simulink model "demo"  (R2021b)
settings: Solver=VariableStepAuto  StartTime=0.0  StopTime=10  RelTol=1e-3
undefined symbols (not defined in the file or in its folder): xc7vx485tffg1157
libraries: hdlBasic x1736, vmcUtilities x1
(part 7 of 7)

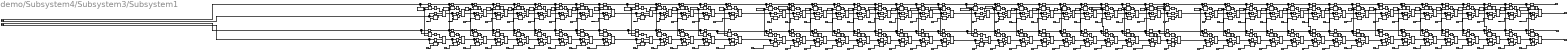
== system demo/Subsystem4/Subsystem3/Subsystem1 ==
  note: 50
  note: 80
  note: 70
  note: 60
  note: 40
  In1 : Inport
  In2 : Inport  Port=2
  In3 : Inport  Port=3
  In4 : Inport  Port=4
  In5 : Inport  Port=5
  In6 : Inport  Port=6
  In7 : Inport  Port=7
  In8 : Inport  Port=8
  In9 : Inport  Port=9
  In10 : Inport  Port=10
  In11 : Inport  Port=11
  In12 : Inport  Port=12
  In13 : Inport  Port=13
  In14 : Inport  Port=14
  In15 : Inport  Port=15
  In16 : Inport  Port=16
  In17 : Inport  Port=17
  In18 : Inport  Port=18
  In19 : Inport  Port=19
  In20 : Inport  Port=20
  In21 : Inport  Port=21
  In22 : Inport  Port=22
  In23 : Inport  Port=23
  In24 : Inport  Port=24
  In25 : Inport  Port=25
  In26 : Inport  Port=26
  In27 : Inport  Port=27
  In28 : Inport  Port=28
  In29 : Inport  Port=29
  In30 : Inport  Port=30
  In31 : Inport  Port=31
  In32 : Inport  Port=32
  In33 : Inport  Port=33
  In34 : Inport  Port=34
  In35 : Inport  Port=35
  In36 : Inport  Port=36
  In37 : Inport  Port=37
  In38 : Inport  Port=38
  In39 : Inport  Port=39
  In40 : Inport  Port=40
  In41 : Inport  Port=41
  In42 : Inport  Port=42
  In43 : Inport  Port=43
  In44 : Inport  Port=44
  In45 : Inport  Port=45
  In46 : Inport  Port=46
  In47 : Inport  Port=47
  In48 : Inport  Port=48
  In49 : Inport  Port=49
  In50 : Inport  Port=50
  In51 : Inport  Port=51
  In52 : Inport  Port=52
  In53 : Inport  Port=53
  In54 : Inport  Port=54
  In55 : Inport  Port=55
  In56 : Inport  Port=56
  In57 : Inport  Port=57
  In58 : Inport  Port=58
  In59 : Inport  Port=59
  In60 : Inport  Port=60
  In61 : Inport  Port=61
  In62 : Inport  Port=62
  In63 : Inport  Port=63
  In64 : Inport  Port=64
  In65 : Inport  Port=65
  In66 : Inport  Port=66
  In67 : Inport  Port=67
  In68 : Inport  Port=68
  In69 : Inport  Port=69
  In70 : Inport  Port=70
  In71 : Inport  Port=71
  In72 : Inport  Port=72
  In73 : Inport  Port=73
  In74 : Inport  Port=74
  In75 : Inport  Port=75
  In76 : Inport  Port=76
  In77 : Inport  Port=77
  In78 : Inport  Port=78
  In79 : Inport  Port=79
  In80 : Inport  Port=80
  In81 : Inport  Port=81
  In82 : Inport  Port=82
  In83 : Inport  Port=83
  In84 : Inport  Port=84
  In85 : Inport  Port=85
  In86 : Inport  Port=86
  In87 : Inport  Port=87
  In88 : Inport  Port=88
  In89 : Inport  Port=89
  In90 : Inport  Port=90
  In91 : Inport  Port=91
  In92 : Inport  Port=92
  In93 : Inport  Port=93
  In94 : Inport  Port=94
  In95 : Inport  Port=95
  In96 : Inport  Port=96
  In97 : Inport  Port=97
  In98 : Inport  Port=98
  In99 : Inport  Port=99
  In100 : Inport  Port=100
  In101 : Inport  Port=101
  In102 : Inport  Port=102
  AddSub{39..40,62..69,80..86,88..95,98..101,103,105..107,109,112,114..137,139,141..163,172..183,191,194,201} (98 alike) : hdlBasic/AddSub  mode=Addition  use_carryin=off  use_carryout=off  en=off  latency=1  precision=User Defined  arith_type="Signed  (2's comp)"  n_bits=32  bin_pt=0  quantization=Truncate  overflow=Wrap  use_behavioral_HDL=off  hw_selection=Fabric  pipelined=off  XmcBlockStatus=1  maskContainerNames=tabcontainer1  block_type=addsub  block_config=sysgen:Addsub_config
  Delay{110..113,177..180,182..184,186,191..192,195..196,199..200,202..204,207,209..214,217..218,220..221,224..226,229,235..236,239..240,242..243,245,247..248,251..255,293,295..296,298..299,302..303,305..306,308..309,311..313,315..316,318..319,323..324,326..327,329..330,332..333,335..338,340,342..343,345..347,350..351,353..354,357..358,360..362,364..365,367..369,371..373,375..376,379..380,383..384,386..387,389,402..404,409,413,419,429,433..434,437,446,448..449,451..453,455..456,458..459,461,463,465..466,468..469,472..474,476..477,479..480,482..485,487,506,517,519,531..532,534..535,538..539,541..542,544..545,548..550,553..554,556..558,560..561,563..564,566,568..569,571..572,574..575,578..580,582..583,585..586,588,590..591,593..594,596..597} (196 alike) : hdlBasic/Delay  rst=off  en=off  latency=1  reg_retiming=off  XmcBlockStatus=1  maskContainerNames=group1  block_type=delay  block_config=sysgen:Delay_config
  Delay{181,185,190,193,201,206,215,219,222..223,228,230,237,241,244,246,250,294,297,300..301,304,307,310,314,317,320,322,325,328,331,334,339,341,344,348..349,352,355..356,359,363,366,370,374,377..378,381..382,385,388,393,401,422,425,439,445,447,450,454,457,460,462,464,467,470..471,475,478,481,486,495,528,533,536..537,540,543,546..547,551..552,555,559,562,565,567,570,573,576..577,581,584,587,589,592,595,598} (98 alike) : hdlBasic/Delay  rst=off  en=off  latency=2  reg_retiming=off  XmcBlockStatus=1  maskContainerNames=group1  block_type=delay  block_config=sysgen:Delay_config
  Mux{38..39,58..67,78..85,87..92,95..96,98..105,110..117,119..136,139..158,161,170..180,183,190,194,198} (98 alike) : hdlBasic/Mux  inputs=2  en=off  latency=1  precision=Full  arith_type=Unsigned  n_bits=16  bin_pt=14  quantization=Truncate  overflow=Wrap  XmcBlockStatus=1  maskContainerNames=tabcontainer1  block_type=mux  block_config=sysgen:Mux_config
  Relational{37..38,60..69,79..85,87..92,95..96,98..100,102..106,111..118,120..122,124..137,140..163,174..183,185,192,196,201} (98 alike) : hdlBasic/Relational  mode=a>=b  op_type=Bool  en=off  latency=1  XmcBlockStatus=1  maskContainerNames=tabcontainer1  block_type=relational  block_config=sysgen:Relational_config
  logi_b36 : hdlBasic/Constant  const=-0.4193548387096773799598281584621872752904891967773437500  gui_display_data_type=Floating-point  arith_type=Floating-point  n_bits=8  bin_pt=8  preci_type=Double  exp_width=8  frac_width=24  explicit_period=on  period=1  XmcBlockStatus=1  maskContainerNames=tabcontainer1  block_type=constant  block_config=sysgen:Constant_config
  logi_b37 : hdlBasic/Constant  const=-0.4032258064516128781562542826577555388212203979492187500  gui_display_data_type=Floating-point  arith_type=Floating-point  n_bits=8  bin_pt=8  preci_type=Double  exp_width=8  frac_width=24  explicit_period=on  period=1  XmcBlockStatus=1  maskContainerNames=tabcontainer1  block_type=constant  block_config=sysgen:Constant_config
  logi_b38 : hdlBasic/Constant  const=-0.3870967741935483763526804068533238023519515991210937500  gui_display_data_type=Floating-point  arith_type=Floating-point  n_bits=8  bin_pt=8  preci_type=Double  exp_width=8  frac_width=24  explicit_period=on  period=1  XmcBlockStatus=1  maskContainerNames=tabcontainer1  block_type=constant  block_config=sysgen:Constant_config
  logi_b39 : hdlBasic/Constant  const=-0.3709677419354838745491065310488920658826828002929687500  gui_display_data_type=Floating-point  arith_type=Floating-point  n_bits=8  bin_pt=8  preci_type=Double  exp_width=8  frac_width=24  explicit_period=on  period=1  XmcBlockStatus=1  maskContainerNames=tabcontainer1  block_type=constant  block_config=sysgen:Constant_config
  logi_b40 : hdlBasic/Constant  const=-0.3548387096774193727455326552444603294134140014648437500  gui_display_data_type=Floating-point  arith_type=Floating-point  n_bits=8  bin_pt=8  preci_type=Double  exp_width=8  frac_width=24  explicit_period=on  period=1  XmcBlockStatus=1  maskContainerNames=tabcontainer1  block_type=constant  block_config=sysgen:Constant_config
  logi_b41 : hdlBasic/Constant  const=-0.3387096774193548154308075481822015717625617980957031250  gui_display_data_type=Floating-point  arith_type=Floating-point  n_bits=8  bin_pt=8  preci_type=Double  exp_width=8  frac_width=24  explicit_period=on  period=1  XmcBlockStatus=1  maskContainerNames=tabcontainer1  block_type=constant  block_config=sysgen:Constant_config
  logi_b42 : hdlBasic/Constant  const=-0.3225806451612903136272336723777698352932929992675781250  gui_display_data_type=Floating-point  arith_type=Floating-point  n_bits=8  bin_pt=8  preci_type=Double  exp_width=8  frac_width=24  explicit_period=on  period=1  XmcBlockStatus=1  maskContainerNames=tabcontainer1  block_type=constant  block_config=sysgen:Constant_config
  logi_b43 : hdlBasic/Constant  const=-0.3064516129032258118236597965733380988240242004394531250  gui_display_data_type=Floating-point  arith_type=Floating-point  n_bits=8  bin_pt=8  preci_type=Double  exp_width=8  frac_width=24  explicit_period=on  period=1  XmcBlockStatus=1  maskContainerNames=tabcontainer1  block_type=constant  block_config=sysgen:Constant_config
  logi_b44 : hdlBasic/Constant  const=-0.2903225806451612545089346895110793411731719970703125000  gui_display_data_type=Floating-point  arith_type=Floating-point  n_bits=8  bin_pt=8  preci_type=Double  exp_width=8  frac_width=24  explicit_period=on  period=1  XmcBlockStatus=1  maskContainerNames=tabcontainer1  block_type=constant  block_config=sysgen:Constant_config
  logi_b45 : hdlBasic/Constant  const=-0.2741935483870967527053608137066476047039031982421875000  gui_display_data_type=Floating-point  arith_type=Floating-point  n_bits=8  bin_pt=8  preci_type=Double  exp_width=8  frac_width=24  explicit_period=on  period=1  XmcBlockStatus=1  maskContainerNames=tabcontainer1  block_type=constant  block_config=sysgen:Constant_config
  logi_b46 : hdlBasic/Constant  const=-0.2580645161290322509017869379022158682346343994140625000  gui_display_data_type=Floating-point  arith_type=Floating-point  n_bits=8  bin_pt=8  preci_type=Double  exp_width=8  frac_width=24  explicit_period=on  period=1  XmcBlockStatus=1  maskContainerNames=tabcontainer1  block_type=constant  block_config=sysgen:Constant_config
  logi_b47 : hdlBasic/Constant  const=-0.2419354838709677490982130620977841317653656005859375000  gui_display_data_type=Floating-point  arith_type=Floating-point  n_bits=8  bin_pt=8  preci_type=Double  exp_width=8  frac_width=24  explicit_period=on  period=1  XmcBlockStatus=1  maskContainerNames=tabcontainer1  block_type=constant  block_config=sysgen:Constant_config
  logi_b48 : hdlBasic/Constant  const=-0.2258064516129032195390635706644388847053050994873046875  gui_display_data_type=Floating-point  arith_type=Floating-point  n_bits=8  bin_pt=8  preci_type=Double  exp_width=8  frac_width=24  explicit_period=on  period=1  XmcBlockStatus=1  maskContainerNames=tabcontainer1  block_type=constant  block_config=sysgen:Constant_config
  logi_b49 : hdlBasic/Constant  const=-0.2096774193548386899799140792310936376452445983886718750  gui_display_data_type=Floating-point  arith_type=Floating-point  n_bits=8  bin_pt=8  preci_type=Double  exp_width=8  frac_width=24  explicit_period=on  period=1  XmcBlockStatus=1  maskContainerNames=tabcontainer1  block_type=constant  block_config=sysgen:Constant_config
  logi_b50 : hdlBasic/Constant  const=-0.1935483870967741881763402034266619011759757995605468750  gui_display_data_type=Floating-point  arith_type=Floating-point  n_bits=8  bin_pt=8  preci_type=Double  exp_width=8  frac_width=24  explicit_period=on  period=1  XmcBlockStatus=1  maskContainerNames=tabcontainer1  block_type=constant  block_config=sysgen:Constant_config
  logi_b51 : hdlBasic/Constant  const=-0.1774193548387096863727663276222301647067070007324218750  gui_display_data_type=Floating-point  arith_type=Floating-point  n_bits=8  bin_pt=8  preci_type=Double  exp_width=8  frac_width=24  explicit_period=on  period=1  XmcBlockStatus=1  maskContainerNames=tabcontainer1  block_type=constant  block_config=sysgen:Constant_config
  logi_b52 : hdlBasic/Constant  const=-0.1612903225806451568136168361888849176466464996337890625  gui_display_data_type=Floating-point  arith_type=Floating-point  n_bits=8  bin_pt=8  preci_type=Double  exp_width=8  frac_width=24  explicit_period=on  period=1  XmcBlockStatus=1  maskContainerNames=tabcontainer1  block_type=constant  block_config=sysgen:Constant_config
  logi_b53 : hdlBasic/Constant  const=-0.1451612903225806272544673447555396705865859985351562500  gui_display_data_type=Floating-point  arith_type=Floating-point  n_bits=8  bin_pt=8  preci_type=Double  exp_width=8  frac_width=24  explicit_period=on  period=1  XmcBlockStatus=1  maskContainerNames=tabcontainer1  block_type=constant  block_config=sysgen:Constant_config
  logi_b54 : hdlBasic/Constant  const=-0.1290322580645161254508934689511079341173171997070312500  gui_display_data_type=Floating-point  arith_type=Floating-point  n_bits=8  bin_pt=8  preci_type=Double  exp_width=8  frac_width=24  explicit_period=on  period=1  XmcBlockStatus=1  maskContainerNames=tabcontainer1  block_type=constant  block_config=sysgen:Constant_config
  logi_b55 : hdlBasic/Constant  const=-0.1129032258064516097695317853322194423526525497436523438  gui_display_data_type=Floating-point  arith_type=Floating-point  n_bits=8  bin_pt=8  preci_type=Double  exp_width=8  frac_width=24  explicit_period=on  period=1  XmcBlockStatus=1  maskContainerNames=tabcontainer1  block_type=constant  block_config=sysgen:Constant_config
  logi_b56 : hdlBasic/Constant  const=-0.0967741935483870940881701017133309505879878997802734375  gui_display_data_type=Floating-point  arith_type=Floating-point  n_bits=8  bin_pt=8  preci_type=Double  exp_width=8  frac_width=24  explicit_period=on  period=1  XmcBlockStatus=1  maskContainerNames=tabcontainer1  block_type=constant  block_config=sysgen:Constant_config
  logi_b57 : hdlBasic/Constant  const=-0.0806451612903225784068084180944424588233232498168945312  gui_display_data_type=Floating-point  arith_type=Floating-point  n_bits=8  bin_pt=8  preci_type=Double  exp_width=8  frac_width=24  explicit_period=on  period=1  XmcBlockStatus=1  maskContainerNames=tabcontainer1  block_type=constant  block_config=sysgen:Constant_config
  logi_b58 : hdlBasic/Constant  const=-0.0645161290322580627254467344755539670586585998535156250  gui_display_data_type=Floating-point  arith_type=Floating-point  n_bits=8  bin_pt=8  preci_type=Double  exp_width=8  frac_width=24  explicit_period=on  period=1  XmcBlockStatus=1  maskContainerNames=tabcontainer1  block_type=constant  block_config=sysgen:Constant_config
  logi_b59 : hdlBasic/Constant  const=-0.0483870967741935470440850508566654752939939498901367188  gui_display_data_type=Floating-point  arith_type=Floating-point  n_bits=8  bin_pt=8  preci_type=Double  exp_width=8  frac_width=24  explicit_period=on  period=1  XmcBlockStatus=1  maskContainerNames=tabcontainer1  block_type=constant  block_config=sysgen:Constant_config
  logi_b60 : hdlBasic/Constant  const=-0.0322580645161290313627233672377769835293292999267578125  gui_display_data_type=Floating-point  arith_type=Floating-point  n_bits=8  bin_pt=8  preci_type=Double  exp_width=8  frac_width=24  explicit_period=on  period=1  XmcBlockStatus=1  maskContainerNames=tabcontainer1  block_type=constant  block_config=sysgen:Constant_config
  logi_b61 : hdlBasic/Constant  const=-0.0161290322580645156813616836188884917646646499633789062  gui_display_data_type=Floating-point  arith_type=Floating-point  n_bits=8  bin_pt=8  preci_type=Double  exp_width=8  frac_width=24  explicit_period=on  period=1  XmcBlockStatus=1  maskContainerNames=tabcontainer1  block_type=constant  block_config=sysgen:Constant_config
  logi_b62 : hdlBasic/Constant  const=0.0000000000000000000000000000000000000000000000000000000  gui_display_data_type=Floating-point  arith_type=Floating-point  n_bits=8  bin_pt=8  preci_type=Double  exp_width=8  frac_width=24  explicit_period=on  period=1  XmcBlockStatus=1  maskContainerNames=tabcontainer1  block_type=constant  block_config=sysgen:Constant_config
  logi_b63 : hdlBasic/Constant  const=0.0161290322580645156813616836188884917646646499633789062  gui_display_data_type=Floating-point  arith_type=Floating-point  n_bits=8  bin_pt=8  preci_type=Double  exp_width=8  frac_width=24  explicit_period=on  period=1  XmcBlockStatus=1  maskContainerNames=tabcontainer1  block_type=constant  block_config=sysgen:Constant_config
  logi_b64 : hdlBasic/Constant  const=0.0322580645161290313627233672377769835293292999267578125  gui_display_data_type=Floating-point  arith_type=Floating-point  n_bits=8  bin_pt=8  preci_type=Double  exp_width=8  frac_width=24  explicit_period=on  period=1  XmcBlockStatus=1  maskContainerNames=tabcontainer1  block_type=constant  block_config=sysgen:Constant_config
  logi_b65 : hdlBasic/Constant  const=0.0483870967741935470440850508566654752939939498901367188  gui_display_data_type=Floating-point  arith_type=Floating-point  n_bits=8  bin_pt=8  preci_type=Double  exp_width=8  frac_width=24  explicit_period=on  period=1  XmcBlockStatus=1  maskContainerNames=tabcontainer1  block_type=constant  block_config=sysgen:Constant_config
  logi_b66 : hdlBasic/Constant  const=0.0645161290322580627254467344755539670586585998535156250  gui_display_data_type=Floating-point  arith_type=Floating-point  n_bits=8  bin_pt=8  preci_type=Double  exp_width=8  frac_width=24  explicit_period=on  period=1  XmcBlockStatus=1  maskContainerNames=tabcontainer1  block_type=constant  block_config=sysgen:Constant_config
  logi_b67 : hdlBasic/Constant  const=0.0806451612903225784068084180944424588233232498168945312  gui_display_data_type=Floating-point  arith_type=Floating-point  n_bits=8  bin_pt=8  preci_type=Double  exp_width=8  frac_width=24  explicit_period=on  period=1  XmcBlockStatus=1  maskContainerNames=tabcontainer1  block_type=constant  block_config=sysgen:Constant_config
  logi_b68 : hdlBasic/Constant  const=0.0967741935483870940881701017133309505879878997802734375  gui_display_data_type=Floating-point  arith_type=Floating-point  n_bits=8  bin_pt=8  preci_type=Double  exp_width=8  frac_width=24  explicit_period=on  period=1  XmcBlockStatus=1  maskContainerNames=tabcontainer1  block_type=constant  block_config=sysgen:Constant_config
  logi_b69 : hdlBasic/Constant  const=0.1129032258064516097695317853322194423526525497436523438  gui_display_data_type=Floating-point  arith_type=Floating-point  n_bits=8  bin_pt=8  preci_type=Double  exp_width=8  frac_width=24  explicit_period=on  period=1  XmcBlockStatus=1  maskContainerNames=tabcontainer1  block_type=constant  block_config=sysgen:Constant_config
  logi_b70 : hdlBasic/Constant  const=0.1290322580645161254508934689511079341173171997070312500  gui_display_data_type=Floating-point  arith_type=Floating-point  n_bits=8  bin_pt=8  preci_type=Double  exp_width=8  frac_width=24  explicit_period=on  period=1  XmcBlockStatus=1  maskContainerNames=tabcontainer1  block_type=constant  block_config=sysgen:Constant_config
  logi_b71 : hdlBasic/Constant  const=0.1451612903225806272544673447555396705865859985351562500  gui_display_data_type=Floating-point  arith_type=Floating-point  n_bits=8  bin_pt=8  preci_type=Double  exp_width=8  frac_width=24  explicit_period=on  period=1  XmcBlockStatus=1  maskContainerNames=tabcontainer1  block_type=constant  block_config=sysgen:Constant_config
  logi_b72 : hdlBasic/Constant  const=0.1612903225806451568136168361888849176466464996337890625  gui_display_data_type=Floating-point  arith_type=Floating-point  n_bits=8  bin_pt=8  preci_type=Double  exp_width=8  frac_width=24  explicit_period=on  period=1  XmcBlockStatus=1  maskContainerNames=tabcontainer1  block_type=constant  block_config=sysgen:Constant_config
  logi_b73 : hdlBasic/Constant  const=0.1774193548387096863727663276222301647067070007324218750  gui_display_data_type=Floating-point  arith_type=Floating-point  n_bits=8  bin_pt=8  preci_type=Double  exp_width=8  frac_width=24  explicit_period=on  period=1  XmcBlockStatus=1  maskContainerNames=tabcontainer1  block_type=constant  block_config=sysgen:Constant_config
  logi_b74 : hdlBasic/Constant  const=0.1935483870967741881763402034266619011759757995605468750  gui_display_data_type=Floating-point  arith_type=Floating-point  n_bits=8  bin_pt=8  preci_type=Double  exp_width=8  frac_width=24  explicit_period=on  period=1  XmcBlockStatus=1  maskContainerNames=tabcontainer1  block_type=constant  block_config=sysgen:Constant_config
  logi_b75 : hdlBasic/Constant  const=0.2096774193548386899799140792310936376452445983886718750  gui_display_data_type=Floating-point  arith_type=Floating-point  n_bits=8  bin_pt=8  preci_type=Double  exp_width=8  frac_width=24  explicit_period=on  period=1  XmcBlockStatus=1  maskContainerNames=tabcontainer1  block_type=constant  block_config=sysgen:Constant_config
  logi_b76 : hdlBasic/Constant  const=0.2258064516129032195390635706644388847053050994873046875  gui_display_data_type=Floating-point  arith_type=Floating-point  n_bits=8  bin_pt=8  preci_type=Double  exp_width=8  frac_width=24  explicit_period=on  period=1  XmcBlockStatus=1  maskContainerNames=tabcontainer1  block_type=constant  block_config=sysgen:Constant_config
  logi_b77 : hdlBasic/Constant  const=0.2419354838709677490982130620977841317653656005859375000  gui_display_data_type=Floating-point  arith_type=Floating-point  n_bits=8  bin_pt=8  preci_type=Double  exp_width=8  frac_width=24  explicit_period=on  period=1  XmcBlockStatus=1  maskContainerNames=tabcontainer1  block_type=constant  block_config=sysgen:Constant_config
  logi_b78 : hdlBasic/Constant  const=0.2580645161290322509017869379022158682346343994140625000  gui_display_data_type=Floating-point  arith_type=Floating-point  n_bits=8  bin_pt=8  preci_type=Double  exp_width=8  frac_width=24  explicit_period=on  period=1  XmcBlockStatus=1  maskContainerNames=tabcontainer1  block_type=constant  block_config=sysgen:Constant_config
  logi_b79 : hdlBasic/Constant  const=0.2741935483870967527053608137066476047039031982421875000  gui_display_data_type=Floating-point  arith_type=Floating-point  n_bits=8  bin_pt=8  preci_type=Double  exp_width=8  frac_width=24  explicit_period=on  period=1  XmcBlockStatus=1  maskContainerNames=tabcontainer1  block_type=constant  block_config=sysgen:Constant_config
  logi_b80 : hdlBasic/Constant  const=0.2903225806451612545089346895110793411731719970703125000  gui_display_data_type=Floating-point  arith_type=Floating-point  n_bits=8  bin_pt=8  preci_type=Double  exp_width=8  frac_width=24  explicit_period=on  period=1  XmcBlockStatus=1  maskContainerNames=tabcontainer1  block_type=constant  block_config=sysgen:Constant_config
  logi_b81 : hdlBasic/Constant  const=0.3064516129032258118236597965733380988240242004394531250  gui_display_data_type=Floating-point  arith_type=Floating-point  n_bits=8  bin_pt=8  preci_type=Double  exp_width=8  frac_width=24  explicit_period=on  period=1  XmcBlockStatus=1  maskContainerNames=tabcontainer1  block_type=constant  block_config=sysgen:Constant_config
  logi_b82 : hdlBasic/Constant  const=0.3225806451612903136272336723777698352932929992675781250  gui_display_data_type=Floating-point  arith_type=Floating-point  n_bits=8  bin_pt=8  preci_type=Double  exp_width=8  frac_width=24  explicit_period=on  period=1  XmcBlockStatus=1  maskContainerNames=tabcontainer1  block_type=constant  block_config=sysgen:Constant_config
  logi_b83 : hdlBasic/Constant  const=0.3387096774193548154308075481822015717625617980957031250  gui_display_data_type=Floating-point  arith_type=Floating-point  n_bits=8  bin_pt=8  preci_type=Double  exp_width=8  frac_width=24  explicit_period=on  period=1  XmcBlockStatus=1  maskContainerNames=tabcontainer1  block_type=constant  block_config=sysgen:Constant_config
  logi_b84 : hdlBasic/Constant  const=0.3548387096774193727455326552444603294134140014648437500  gui_display_data_type=Floating-point  arith_type=Floating-point  n_bits=8  bin_pt=8  preci_type=Double  exp_width=8  frac_width=24  explicit_period=on  period=1  XmcBlockStatus=1  maskContainerNames=tabcontainer1  block_type=constant  block_config=sysgen:Constant_config
  Out1 : Outport
  Out2 : Outport  Port=2
  Out3 : Outport  Port=3
  Out4 : Outport  Port=4
  wires:
  In12/1 -> AddSub86/2
  Delay361/1 -> Mux154/1
  Delay112/1 -> Mux38/1
  Delay590/1 -> Mux115/1
  Delay384/1 -> Mux147/2
  Delay213/1 -> Mux111/2
  AddSub67/1 -> Mux65/3
  Delay329/1 -> Mux78/1
  Relational135/1 -> Delay571/1
  Relational113/1 -> Delay582/1
  AddSub131/1 -> Mux129/3
  Delay245/1 -> Mux194/2
  Delay313/1 -> Mux63/2
  Relational117/1 -> Delay596/1
  AddSub112/1 -> Mux59/3
  Delay326/1 -> Mux67/1
  In71/1 -> AddSub95/2
  Relational102/1 -> Delay448/1
  Delay368/1 -> Mux156/2
  Delay531/1 -> Mux121/1
  Relational79/1 -> Delay295/1
  Relational196/1 -> Delay473/1
  Relational112/1 -> Delay224/1
  Mux131/1 -> AddSub132/1, Delay564/1
  Mux116/1 -> AddSub131/1, Delay597/1
  Delay382/1 -> Delay393/1, Relational163/1
  Relational131/1 -> Delay548/1
  logi_b66/1 -> Relational120/2, Relational137/2
  Mux61/1 -> AddSub91/1, Delay218/1
  Mux140/1 -> Delay333/1, AddSub145/1
  Delay336/1 -> Mux96/1
  Delay462/1 -> Relational122/1, Delay495/1
  Mux65/1 -> AddSub68/1, Delay324/1
  logi_b37/1 -> Relational62/2, Relational68/2
  Delay306/1 -> Mux83/2
  logi_b72/1 -> Relational148/2, Relational156/2
  logi_b83/1 -> Relational183/2, Relational106/2
  Relational201/1 -> Delay433/1
  In49/1 -> AddSub132/2
  Delay593/1 -> Mux116/1
  In2/1 -> Delay184/1, AddSub112/1
  Delay349/1 -> Relational152/1, Delay382/1
  Delay542/1 -> Mux124/2
  AddSub151/1 -> Mux147/3
  Relational158/1 -> Delay364/1
  Delay569/1 -> Mux133/2
  logi_b58/1 -> Relational98/2, Relational122/2
  Delay315/1 -> Mux64/1
  Delay479/1 -> Mux177/1
  Delay482/1 -> Mux178/1
  Mux141/1 -> Delay337/1, AddSub162/1
  In8/1 -> AddSub109/2
  In20/1 -> AddSub100/2
  AddSub162/1 -> Mux96/3
  logi_b40/1 -> Relational65/2, Relational81/2
  AddSub114/1 -> Mux111/3
  Delay301/1 -> Delay304/1, Relational82/1
  logi_b45/1 -> Relational89/2, Relational88/2
  Delay583/1 -> Mux113/2
  Delay214/1 -> Mux61/2
  AddSub105/1 -> Mux131/3
  In30/1 -> AddSub101/2
  Delay447/1 -> Delay450/1, Relational103/1
  Mux62/1 -> AddSub65/1, Delay313/1
  AddSub128/1 -> Mux139/3
  Relational82/1 -> Delay305/1
  In22/1 -> AddSub172/2
  Mux80/1 -> AddSub81/1, Delay299/1
  Delay439/1 -> Relational196/1, Delay462/1
  Mux98/1 -> AddSub100/1, Delay221/1
  logi_b43/1 -> Relational69/2, Relational84/2
  Delay222/1 -> Delay547/1, Relational37/1
  AddSub159/1 -> Mux157/3
  Delay203/1 -> Mux58/1
  Delay592/1 -> Delay595/1, Relational117/1
  Delay314/1 -> Relational63/1, Delay317/1
  Delay481/1 -> Relational162/1, Delay486/1
  Delay464/1 -> Relational177/1, Delay467/1
  AddSub129/1 -> Mux126/3
  Delay218/1 -> Mux98/2
  Mux88/1 -> Delay204/1, AddSub109/1
  Relational181/1 -> Delay479/1
  Relational160/1 -> Delay345/1
  Delay344/1 -> Delay464/1, Relational176/1
  Mux66/1 -> AddSub69/1, Delay327/1
  Delay594/1 -> Mux116/2
  Relational149/1 -> Delay383/1
  Relational114/1 -> Delay585/1
  AddSub121/1 -> Mux119/3
  Relational174/1 -> Delay429/1
  AddSub173/1 -> Mux180/3
  Delay551/1 -> Relational111/1, Delay223/1
  Delay571/1 -> Mux134/1
  logi_b39/1 -> Relational64/2, Relational80/2
  Delay300/1 -> Delay301/1, Relational81/1
  Delay486/1 -> Out3/1
  Mux125/1 -> AddSub129/1, Delay549/1
  Delay413/1 -> Mux150/2
  Relational140/1 -> Delay252/1
  AddSub134/1 -> Mux133/3
  Mux110/1 -> AddSub144/1, Delay351/1
  Delay239/1 -> Mux91/1
  Mux177/1 -> AddSub181/1, Delay483/1
  Delay403/1 -> Mux103/2
  Delay589/1 -> Delay592/1, Relational116/1
  logi_b50/1 -> Relational121/2, Relational95/2
  Relational133/1 -> Delay563/1
  Delay595/1 -> Relational120/1, Delay598/1
  Relational62/1 -> Delay182/1
  In34/1 -> AddSub161/2
  In72/1 -> AddSub39/2
  Delay235/1 -> Mux194/1
  Mux123/1 -> AddSub126/1, Delay542/1
  logi_b84/1 -> Relational162/2, Relational175/2
  In57/1 -> AddSub88/2
  Relational68/1 -> Delay186/1
  Mux179/1 -> Out2/1
  Mux87/1 -> Delay200/1, AddSub92/1
  AddSub100/1 -> Mux99/3
  AddSub109/1 -> Mux58/3
  AddSub117/1 -> Mux114/3
  Relational103/1 -> Delay452/1
  Mux58/1 -> AddSub90/1, Delay214/1
  Relational122/1 -> Delay506/1
  AddSub65/1 -> Mux63/3
  Delay355/1 -> Delay356/1, Relational156/1
  In21/1 -> AddSub40/2
  Relational92/1 -> Delay242/1
  AddSub181/1 -> Mux178/3
  Delay251/1 -> Mux128/1
  AddSub126/1 -> Mux124/3
  Delay365/1 -> Mux155/2
  AddSub148/1 -> Mux145/3
  Delay337/1 -> Mux96/2
  Delay434/1 -> Mux161/2
  Delay113/1 -> Mux38/2
  Delay199/1 -> Mux89/1
  Delay409/1 -> Mux180/1
  Delay597/1 -> Mux129/2
  Relational80/1 -> Delay298/1
  logi_b77/1 -> Relational176/2, Relational182/2
  AddSub176/1 -> Mux174/3
  Delay200/1 -> Mux89/2
  Delay110/1 -> Mux39/1
  Delay574/1 -> Mux135/1
  AddSub98/1 -> Mux95/3
  logi_b74/1 -> Relational150/2, Relational158/2
  logi_b44/1 -> Relational85/2, Relational87/2
  AddSub172/1 -> Mux183/3
  In98/1 -> AddSub117/2
  AddSub135/1 -> Mux134/3
  Delay206/1 -> Delay215/1, Relational96/1
  In90/1 -> AddSub118/2
  AddSub141/1 -> Mux140/3
  Delay554/1 -> Mux119/2
  Relational180/1 -> Delay476/1
  Delay372/1 -> Mux144/1
  Mux114/1 -> AddSub118/1, Delay591/1
  Delay331/1 -> Relational85/1, Delay193/1
  Delay202/1 -> Mux90/1
  Delay250/1 -> Relational144/1, Delay334/1
  Mux143/1 -> AddSub147/1, Delay373/1
  Delay577/1 -> Relational130/1, Delay230/1
  In46/1 -> AddSub120/2
  AddSub174/1 -> Mux171/3
  Delay332/1 -> Mux142/1
  Mux95/1 -> AddSub99/1, Delay209/1
  Delay584/1 -> Relational114/1, Delay587/1
  Delay586/1 -> Mux114/2
  In80/1 -> AddSub129/2
  Mux153/1 -> AddSub156/1, Delay362/1
  In38/1 -> AddSub156/2
  AddSub132/1 -> Mux132/3
  Mux161/1 -> AddSub161/1, Delay451/1
  AddSub139/1 -> Mux150/3
  Delay453/1 -> Mux100/2
  Mux124/1 -> AddSub127/1, Delay545/1
  Delay244/1 -> Relational38/1, Delay552/1
  In62/1 -> AddSub68/2
  Delay246/1 -> Relational143/1, Delay339/1
  AddSub158/1 -> Mux156/3
  logi_b82/1 -> Relational181/2, Relational104/2
  logi_b69/1 -> Relational145/2, Relational151/2
  Mux135/1 -> AddSub137/1, Delay579/1
  Delay560/1 -> Mux131/1
  Delay575/1 -> Mux135/2
  Mux83/1 -> AddSub85/1, Delay309/1
  Relational146/1 -> Delay372/1
  Mux112/1 -> AddSub116/1, Delay583/1
  Mux127/1 -> Delay226/1, AddSub194/1
  Delay598/1 -> Relational140/1, Delay250/1
  Mux81/1 -> AddSub83/1, Delay303/1
  Delay325/1 -> Delay328/1, Relational67/1
  Relational106/1 -> Delay458/1
  logi_b80/1 -> Relational179/2, Relational102/2
  Delay506/1 -> Mux127/1
  AddSub149/1 -> Mux146/3
  Delay327/1 -> Mux67/2
  Delay219/1 -> Relational100/1, Delay222/1
  Delay385/1 -> Relational153/1, Delay388/1
  In43/1 -> AddSub155/2
  In7/1 -> AddSub62/2
  Delay353/1 -> Mux152/1
  Delay587/1 -> Delay589/1, Relational115/1
  Delay561/1 -> Mux131/2
  In11/1 -> AddSub85/2
  Relational185/1 -> Delay446/1
  Delay322/1 -> Delay325/1, Relational66/1
  Delay581/1 -> Relational113/1, Delay584/1
  In51/1 -> AddSub153/2
  Mux174/1 -> AddSub177/1, Delay474/1
  Mux113/1 -> AddSub117/1, Delay586/1
  Delay335/1 -> Mux143/1
  In56/1 -> AddSub82/2
  logi_b68/1 -> Relational144/2, Relational143/2
  Delay483/1 -> Mux178/2
  In9/1 -> AddSub90/2
  AddSub90/1 -> Mux61/3
  Delay573/1 -> Relational137/1, Delay576/1
  In14/1 -> AddSub103/2
  Mux64/1 -> AddSub67/1, Delay319/1
  In73/1 -> AddSub121/2
  logi_b46/1 -> Relational90/2, Relational96/2
  Relational61/1 -> Delay179/1
  In41/1 -> AddSub139/2
  logi_b62/1 -> Relational114/2, Relational133/2
  Delay422/1 -> Delay439/1, Relational185/1
  Delay341/1 -> Delay401/1, Relational182/1
  Delay539/1 -> Mux123/2
  Relational143/1 -> Delay336/1
  Delay317/1 -> Relational64/1, Delay320/1
  Delay333/1 -> Mux142/2
  AddSub88/1 -> Mux87/3
  logi_b48/1 -> Relational92/2, Relational100/2
  Delay375/1 -> Mux145/1
  Relational84/1 -> Delay311/1
  Relational38/1 -> Delay112/1
  In42/1 -> AddSub134/2
  In39/1 -> AddSub157/2
  In102/1 -> AddSub148/2
  logi_b56/1 -> Relational129/2, Relational185/2
  AddSub183/1 -> Mux194/3
  logi_b54/1 -> Relational127/2, Relational163/2
  In6/1 -> AddSub112/2
  In58/1 -> AddSub178/2
  Relational152/1 -> Delay360/1
  AddSub68/1 -> Mux66/3
  Delay351/1 -> Mux151/2
  Relational85/1 -> Delay195/1
  AddSub150/1 -> Mux161/3
  Mux39/1 -> Delay566/1, AddSub98/1
  In60/1 -> AddSub181/2
  In77/1 -> AddSub176/2
  Delay465/1 -> Mux173/1
  In96/1 -> AddSub115/2
  Mux152/1 -> AddSub155/1, Delay358/1
  Delay111/1 -> Mux39/2
  In25/1 -> AddSub160/2
  Mux170/1 -> AddSub173/1, Delay419/1
  Delay459/1 -> Mux102/2
  In84/1 -> AddSub133/2
  Delay550/1 -> Mux127/2
  Mux151/1 -> AddSub153/1, Delay354/1
  Delay297/1 -> Relational80/1, Delay300/1
  Delay253/1 -> Mux140/2
  Delay389/1 -> Mux170/2
  Delay495/1 -> Relational105/1, Delay228/1
  Delay377/1 -> Delay378/1, Relational148/1
  Delay298/1 -> Mux81/1
  Delay556/1 -> Mux120/1
  In35/1 -> AddSub135/2
  AddSub137/1 -> Mux136/3
  Mux149/1 -> AddSub159/1, Delay346/1
  Delay477/1 -> Mux176/2
  Relational163/1 -> Delay404/1
  Relational148/1 -> Delay379/1
  Mux92/1 -> AddSub39/1, Delay113/1
  In89/1 -> AddSub125/2
  Delay220/1 -> Mux99/1
  Relational63/1 -> Delay315/1
  AddSub178/1 -> Mux176/3
  AddSub136/1 -> Mux135/3
  In44/1 -> AddSub98/2
  Relational64/1 -> Delay318/1
  Delay180/1 -> Mux62/2
  In92/1 -> AddSub122/2
  Relational95/1 -> Delay557/1
  Relational156/1 -> Delay357/1
  In13/1 -> AddSub201/2
  Delay472/1 -> Mux175/1
  Delay196/1 -> Mux87/2
  Mux172/1 -> AddSub172/1, Delay484/1
  Relational151/1 -> Delay340/1
  Delay461/1 -> Mux179/1
  Mux60/1 -> AddSub63/1, Delay296/1
  Relational66/1 -> Delay326/1
  Mux122/1 -> AddSub125/1, Delay539/1
  Delay532/1 -> Mux121/2
  logi_b59/1 -> Relational111/2, Relational105/2
  In5/1 -> AddSub182/2
  Delay404/1 -> Mux150/1
  Delay252/1 -> Mux140/1
  In74/1 -> AddSub159/2
  AddSub82/1 -> Mux79/3
  AddSub94/1 -> Mux91/3
  Delay469/1 -> Mux174/2
  In32/1 -> AddSub143/2
  In78/1 -> AddSub126/2
  AddSub142/1 -> Mux141/3
  Delay562/1 -> Relational133/1, Delay565/1
  Delay241/1 -> Relational92/1, Delay244/1
  In65/1 -> AddSub65/2
  Delay295/1 -> Mux80/1
  logi_b73/1 -> Relational149/2, Relational157/2
  AddSub155/1 -> Mux153/3
  In53/1 -> Delay180/1, AddSub64/1
  AddSub106/1 -> Mux102/3
  Relational127/1 -> Delay538/1
  Mux82/1 -> AddSub84/1, Delay306/1
  Delay540/1 -> Delay543/1, Relational129/1
  logi_b71/1 -> Relational147/2, Relational155/2
  Relational183/1 -> Delay482/1
  logi_b67/1 -> Relational140/2, Relational142/2
  AddSub133/1 -> Mux130/3
  AddSub115/1 -> Mux112/3
  Delay537/1 -> Delay540/1, Relational128/1
  AddSub39/1 -> Mux38/3
  In24/1 -> AddSub142/2
  Delay191/1 -> Mux88/1
  In94/1 -> AddSub124/2
  Delay572/1 -> Mux134/2
  Relational125/1 -> Delay531/1
  In100/1 -> AddSub146/2
  Mux96/1 -> AddSub143/1, Delay347/1
  Delay401/1 -> Relational192/1, Delay425/1
  Mux119/1 -> AddSub122/1, Delay517/1
  Mux130/1 -> AddSub141/1, Delay253/1
  In37/1 -> AddSub137/2
  Mux146/1 -> AddSub151/1, Delay384/1
  Delay545/1 -> Mux125/2
  In1/1 -> Relational60/1, Delay185/1
  Mux190/1 -> AddSub191/1, Delay449/1
  In69/1 -> AddSub93/2
  Delay480/1 -> Mux177/2
  Delay433/1 -> Mux190/1
  Delay237/1 -> Relational91/1, Delay241/1
  In79/1 -> AddSub127/2
  Delay179/1 -> Mux62/1
  Delay183/1 -> Mux59/1
  Delay299/1 -> Mux81/2
  logi_b57/1 -> Relational131/2, Relational196/2
  In15/1 -> AddSub83/2
  Delay582/1 -> Mux113/1
  Delay363/1 -> Relational159/1, Delay366/1
  Delay294/1 -> Relational79/1, Delay297/1
  In91/1 -> AddSub149/2
  Relational111/1 -> Delay212/1
  Delay538/1 -> Mux123/1
  Mux180/1 -> AddSub180/1, Delay437/1
  Relational162/1 -> Delay402/1
  In40/1 -> AddSub158/2
  Delay445/1 -> Delay447/1, Relational102/1
  AddSub152/1 -> Mux148/3
  logi_b63/1 -> Relational115/2, Relational134/2
  AddSub123/1 -> Mux121/3
  Delay476/1 -> Mux176/1
  Delay217/1 -> Mux98/1
  Mux111/1 -> AddSub115/1, Delay580/1
  Mux176/1 -> AddSub179/1, Delay480/1
  Mux67/1 -> AddSub80/1, Delay330/1
  Relational128/1 -> Delay541/1
  Mux103/1 -> Out4/1
  In26/1 -> AddSub163/2
  Relational100/1 -> Delay220/1
  Relational81/1 -> Delay302/1
  Relational182/1 -> Delay519/1
  Delay186/1 -> Mux60/1
  Delay552/1 -> Delay555/1, Relational121/1
  Delay470/1 -> Delay471/1, Relational179/1
  Delay185/1 -> Delay294/1, Relational68/1
  Mux144/1 -> AddSub148/1, Delay376/1
  In76/1 -> AddSub175/2
  Relational60/1 -> Delay183/1
  Delay467/1 -> Relational178/1, Delay470/1
  In68/1 -> AddSub92/2
  Relational175/1 -> Delay461/1
  Delay579/1 -> Mux136/2
  logi_b60/1 -> Relational112/2, Relational118/2
  Delay449/1 -> Mux198/2
  Delay318/1 -> Mux65/1
  Delay568/1 -> Mux133/1
  Delay388/1 -> Relational160/1, Delay344/1
  Relational118/1 -> Delay229/1
  In95/1 -> AddSub114/2
  AddSub119/1 -> Mux116/3
  AddSub201/1 -> Mux100/3
  logi_b55/1 -> Relational128/2, Relational174/2
  Mux100/1 -> AddSub103/1, Delay456/1
  Relational132/1 -> Delay560/1
  Mux120/1 -> AddSub123/1, Delay532/1
  logi_b52/1 -> Relational125/2, Relational141/2
  Relational37/1 -> Delay110/1
  AddSub177/1 -> Mux175/3
  Mux139/1 -> AddSub139/1, Delay413/1
  AddSub99/1 -> Mux117/3
  In63/1 -> AddSub177/2
  Delay309/1 -> Mux84/2
  Delay366/1 -> Relational161/1, Delay341/1
  Mux38/1 -> Delay554/1, AddSub121/1
  Delay316/1 -> Mux64/2
  Relational179/1 -> Delay472/1
  Delay371/1 -> Mux139/2
  In93/1 -> AddSub123/2
  Delay379/1 -> Mux146/1
  In54/1 -> AddSub69/2
  Mux133/1 -> AddSub135/1, Delay572/1
  Mux158/1 -> Delay389/1, AddSub163/1
  logi_b79/1 -> Relational178/2, Relational201/2
  Delay370/1 -> Relational146/1, Delay374/1
  Delay578/1 -> Mux136/1
  Delay254/1 -> Mux149/1
  Delay563/1 -> Mux132/1
  Relational192/1 -> Delay409/1
  Delay310/1 -> Relational87/1, Delay190/1
  In86/1 -> AddSub151/2
  Mux142/1 -> AddSub146/1, Delay369/1
  Delay380/1 -> Mux146/2
  logi_b64/1 -> Relational116/2, Relational135/2
  In99/1 -> AddSub145/2
  In29/1 -> AddSub194/2
  In10/1 -> AddSub84/2
  Mux178/1 -> AddSub107/1, Delay403/1
  AddSub101/1 -> Mux105/3
  AddSub146/1 -> Mux143/3
  Delay182/1 -> Mux63/1
  AddSub143/1 -> Mux110/3
  Delay359/1 -> Delay363/1, Relational158/1
  Delay193/1 -> Relational89/1, Delay201/1
  Mux104/1 -> AddSub101/1, Delay558/1
  Delay455/1 -> Mux101/1
  Delay209/1 -> Mux117/2
  Delay566/1 -> Mux95/2
  AddSub130/1 -> Mux127/3
  Mux84/1 -> AddSub86/1, Delay312/1
  Relational145/1 -> Delay335/1
  Delay352/1 -> Relational155/1, Delay355/1
  Mux91/1 -> AddSub95/1, Delay243/1
  Mux171/1 -> AddSub175/1, Delay466/1
  Delay302/1 -> Mux82/1
  Mux128/1 -> AddSub128/1, Delay371/1
  Relational178/1 -> Delay468/1
  In18/1 -> AddSub81/2
  logi_b36/1 -> Relational61/2, Relational60/2
  Delay362/1 -> Mux154/2
  Mux147/1 -> AddSub152/1, Delay387/1
  Delay345/1 -> Mux157/1
  AddSub95/1 -> Mux92/3
  Delay570/1 -> Delay573/1, Relational136/1
  Relational130/1 -> Delay588/1
  Delay466/1 -> Mux173/2
  Delay369/1 -> Mux143/2
  Delay474/1 -> Mux175/2
  Delay381/1 -> Delay385/1, Relational150/1
  Delay451/1 -> Mux172/2
  Delay457/1 -> Relational175/1, Delay460/1
  Delay484/1 -> Mux183/2
  Delay342/1 -> Mux158/1
  logi_b65/1 -> Relational117/2, Relational136/2
  logi_b47/1 -> Relational91/2, Relational99/2
  Delay215/1 -> Relational99/1, Delay219/1
  AddSub40/1 -> Mux39/3
  Delay450/1 -> Delay454/1, Relational104/1
  Delay533/1 -> Relational126/1, Delay536/1
  Relational141/1 -> Delay251/1
  Mux59/1 -> AddSub62/1, Delay293/1
  Relational116/1 -> Delay593/1
  Relational121/1 -> Delay553/1
  Delay475/1 -> Delay478/1, Relational181/1
  Delay346/1 -> Mux157/2
  Mux78/1 -> AddSub82/1, Delay178/1
  Delay192/1 -> Mux88/2
  Delay374/1 -> Relational147/1, Delay377/1
  AddSub107/1 -> Mux103/3
  AddSub80/1 -> Mux78/3
  Delay541/1 -> Mux124/1
  Mux121/1 -> AddSub124/1, Delay535/1
  logi_b76/1 -> Relational160/2, Relational161/2
  Delay296/1 -> Mux80/2
  Delay181/1 -> Delay314/1, Relational62/1
  In27/1 -> AddSub173/2
  Delay557/1 -> Mux95/1
  Mux155/1 -> AddSub158/1, Delay368/1
  Delay328/1 -> Relational69/1, Delay331/1
  Delay473/1 -> Mux183/1
  Delay446/1 -> Mux172/1
  Delay528/1 -> Relational125/1, Delay533/1
  Delay319/1 -> Mux65/2
  In31/1 -> AddSub162/2
  AddSub182/1 -> Mux179/3
  Delay564/1 -> Mux132/2
  Delay536/1 -> Delay537/1, Relational127/1
  Relational150/1 -> Delay386/1
  Relational136/1 -> Delay574/1
  Mux129/1 -> AddSub133/1, Delay211/1
  AddSub153/1 -> Mux152/3
  Relational154/1 -> Delay350/1
  Delay340/1 -> Mux110/1
  Delay419/1 -> Mux180/2
  Relational161/1 -> Delay342/1
  Delay591/1 -> Mux115/2
  Delay553/1 -> Mux119/1
  Mux136/1 -> AddSub142/1, Delay248/1
  Mux134/1 -> AddSub136/1, Delay575/1
  Delay307/1 -> Relational84/1, Delay310/1
  Mux89/1 -> AddSub93/1, Delay236/1
  Delay312/1 -> Mux85/2
  Mux99/1 -> AddSub40/1, Delay111/1
  Relational155/1 -> Delay353/1
  Mux150/1 -> AddSub150/1, Delay434/1
  AddSub91/1 -> Mux98/3
  Delay429/1 -> Mux161/1
  In59/1 -> AddSub179/2
  Relational65/1 -> Delay323/1
  AddSub125/1 -> Mux123/3
  Delay242/1 -> Mux92/1
  AddSub147/1 -> Mux144/3
  AddSub194/1 -> Mux104/3
  Delay543/1 -> Relational131/1, Delay546/1
  Delay223/1 -> Delay581/1, Relational112/1
  Delay358/1 -> Mux153/2
  Delay305/1 -> Mux83/1
  logi_b49/1 -> Relational38/2, Relational37/2
  Delay225/1 -> Mux104/1
  Delay367/1 -> Mux156/1
  AddSub63/1 -> Mux80/3
  Relational90/1 -> Delay202/1
  Delay184/1 -> Mux59/2
  Mux145/1 -> AddSub149/1, Delay380/1
  Mux154/1 -> AddSub157/1, Delay365/1
  Relational91/1 -> Delay239/1
  Delay559/1 -> Relational132/1, Delay562/1
  Relational124/1 -> Delay556/1
  Mux85/1 -> AddSub89/1, Delay192/1
  Delay195/1 -> Mux87/1
  AddSub93/1 -> Mux90/3
  Delay425/1 -> Relational201/1, Delay445/1
  Delay373/1 -> Mux144/2
  Relational137/1 -> Delay578/1
  Delay311/1 -> Mux85/1
  Delay240/1 -> Mux91/2
  Relational104/1 -> Delay455/1
  Delay463/1 -> Mux171/2
  Relational157/1 -> Delay361/1
  AddSub122/1 -> Mux120/3
  Mux157/1 -> Delay463/1, AddSub174/1
  Mux79/1 -> AddSub88/1, Delay196/1
  AddSub83/1 -> Mux82/3
  Relational67/1 -> Delay329/1
  In70/1 -> AddSub94/2
  AddSub180/1 -> Mux190/3
  logi_b78/1 -> Relational177/2, Relational192/2
  Mux148/1 -> AddSub154/1, Delay255/1
  logi_b42/1 -> Relational67/2, Relational83/2
  logi_b81/1 -> Relational180/2, Relational103/2
  Delay230/1 -> Relational141/1, Delay349/1
  Mux102/1 -> AddSub182/1, Delay485/1
  In48/1 -> AddSub105/2
  Mux173/1 -> AddSub176/1, Delay469/1
  Delay596/1 -> Mux129/1
  Delay364/1 -> Mux155/1
  Delay471/1 -> Delay475/1, Relational180/1
  AddSub124/1 -> Mux122/3
  Relational105/1 -> Delay225/1
  Relational159/1 -> Delay367/1
  Delay226/1 -> Mux104/2
  logi_b61/1 -> Relational113/2, Relational132/2
  In45/1 -> AddSub99/2
  In33/1 -> AddSub150/2
  Delay224/1 -> Mux112/1
  AddSub103/1 -> Mux101/3
  Delay247/1 -> Mux141/1
  Delay478/1 -> Relational183/1, Delay481/1
  In61/1 -> AddSub107/2
  Delay549/1 -> Mux126/2
  Delay378/1 -> Delay381/1, Relational149/1
  AddSub145/1 -> Mux142/3
  AddSub69/1 -> Mux67/3
  Delay565/1 -> Delay567/1, Relational134/1
  Delay393/1 -> Delay422/1, Relational174/1
  Delay576/1 -> Relational142/1, Delay246/1
  logi_b70/1 -> Relational146/2, Relational154/2
  Delay558/1 -> Mux105/2
  Delay320/1 -> Delay322/1, Relational65/1
  Mux115/1 -> AddSub119/1, Delay594/1
  In16/1 -> AddSub191/2
  Delay580/1 -> Mux112/2
  Delay293/1 -> Mux60/2
  Relational153/1 -> Delay254/1
  AddSub81/1 -> Mux81/3
  AddSub120/1 -> Mux128/3
  Delay454/1 -> Relational106/1, Delay457/1
  Delay456/1 -> Mux101/2
  logi_b51/1 -> Relational130/2, Relational124/2
  Delay350/1 -> Mux151/1
  Delay383/1 -> Mux147/1
  Mux198/1 -> AddSub201/1, Delay453/1
  Delay190/1 -> Relational88/1, Delay206/1
  In75/1 -> AddSub174/2
  Delay402/1 -> Mux103/1
  Mux183/1 -> AddSub130/1, Delay550/1
  In4/1 -> AddSub106/2
  Mux132/1 -> AddSub134/1, Delay569/1
  In17/1 -> AddSub63/2
  Delay386/1 -> Mux148/1
  logi_b38/1 -> Relational63/2, Relational79/2
  AddSub118/1 -> Mux115/3
  Delay452/1 -> Mux100/1
  Delay303/1 -> Mux82/2
  AddSub156/1 -> Mux154/3
  Delay544/1 -> Mux125/1
  Delay221/1 -> Mux99/2
  logi_b53/1 -> Relational126/2, Relational152/2
  Delay255/1 -> Mux149/2
  AddSub191/1 -> Mux198/3
  Delay334/1 -> Delay370/1, Relational145/1
  Delay360/1 -> Mux139/1
  In19/1 -> AddSub91/2
  In81/1 -> AddSub183/2
  AddSub163/1 -> Mux170/3
  Relational129/1 -> Delay544/1
  Delay376/1 -> Mux145/2
  Delay212/1 -> Mux111/1
  Relational88/1 -> Delay203/1
  AddSub85/1 -> Mux84/3
  Relational98/1 -> Delay235/1
  Delay356/1 -> Delay359/1, Relational157/1
  Delay228/1 -> Delay559/1, Relational118/1
  Delay343/1 -> Mux158/2
  Delay585/1 -> Mux114/1
  Delay323/1 -> Mux66/1
  In36/1 -> AddSub136/2
  Relational99/1 -> Delay217/1
  Relational134/1 -> Delay568/1
  AddSub154/1 -> Mux149/3
  Relational147/1 -> Delay375/1
  Delay177/1 -> Mux79/1
  Mux175/1 -> AddSub178/1, Delay477/1
  Delay546/1 -> Relational98/1, Delay551/1
  In85/1 -> AddSub141/2
  AddSub160/1 -> Mux158/3
  Delay437/1 -> Mux190/2
  Delay178/1 -> Mux79/2
  Delay354/1 -> Mux152/2
  Delay236/1 -> Mux90/2
  In82/1 -> AddSub119/2
  Relational126/1 -> Delay534/1
  In52/1 -> Relational61/1, Delay181/1
  Delay458/1 -> Mux102/1
  Delay588/1 -> Mux117/1
  Delay339/1 -> Delay348/1, Relational151/1
  Delay567/1 -> Delay570/1, Relational135/1
  Mux101/1 -> AddSub106/1, Delay459/1
  Mux117/1 -> AddSub120/1, Delay338/1
  AddSub175/1 -> Mux173/3
  Delay211/1 -> Mux130/2
  In67/1 -> AddSub67/2
  Delay308/1 -> Mux84/1
  AddSub157/1 -> Mux155/3
  AddSub62/1 -> Mux60/3
  Relational69/1 -> Delay177/1
  Relational115/1 -> Delay590/1
  Delay517/1 -> Mux120/2
  Delay548/1 -> Mux126/1
  AddSub64/1 -> Mux62/3
  logi_b75/1 -> Relational153/2, Relational159/2
  In83/1 -> AddSub131/2
  In101/1 -> AddSub147/2
  In55/1 -> AddSub80/2
  Delay330/1 -> Mux78/2
  AddSub84/1 -> Mux83/3
  In88/1 -> AddSub154/2
  In28/1 -> AddSub180/2
  Mux105/1 -> AddSub105/1, Delay561/1
  Delay207/1 -> Mux61/1
  Mux63/1 -> AddSub66/1, Delay316/1
  Delay243/1 -> Mux92/2
  Relational144/1 -> Delay332/1
  Delay487/1 -> Mux171/1
  Delay387/1 -> Mux148/2
  Delay201/1 -> Delay237/1, Relational90/1
  AddSub179/1 -> Mux177/3
  AddSub127/1 -> Mux125/3
  AddSub161/1 -> Mux172/3
  Delay519/1 -> Mux170/1
  In64/1 -> AddSub64/2
  Delay348/1 -> Relational154/1, Delay352/1
  Relational87/1 -> Delay191/1
  Relational120/1 -> Delay210/1
  In3/1 -> AddSub89/2
  logi_b41/1 -> Relational66/2, Relational82/2
  Delay357/1 -> Mux153/1
  Delay534/1 -> Mux122/1
  Delay547/1 -> Relational95/1, Delay577/1
  Delay324/1 -> Mux66/2
  In23/1 -> AddSub130/2
  Relational89/1 -> Delay199/1
  Delay304/1 -> Delay307/1, Relational83/1
  Delay210/1 -> Mux130/1
  AddSub144/1 -> Mux151/3
  In50/1 -> AddSub144/2
  Delay485/1 -> Mux179/2
  AddSub89/1 -> Mux88/3
  Delay338/1 -> Mux128/2
  Relational83/1 -> Delay308/1
  Delay448/1 -> Mux198/1
  Mux156/1 -> AddSub160/1, Delay343/1
  In66/1 -> AddSub66/2
  Relational177/1 -> Delay465/1
  Relational176/1 -> Delay487/1
  Mux194/1 -> Delay213/1, AddSub114/1
  Mux90/1 -> AddSub94/1, Delay240/1
  AddSub116/1 -> Mux113/3
  Delay460/1 -> Out1/1
  Delay204/1 -> Mux58/2
  In87/1 -> AddSub152/2
  Delay347/1 -> Mux110/2
  Mux126/1 -> AddSub183/1, Delay245/1
  AddSub92/1 -> Mux89/3
  Relational96/1 -> Delay207/1
  In97/1 -> AddSub116/2
  AddSub66/1 -> Mux64/3
  In47/1 -> AddSub128/2
  Relational142/1 -> Delay247/1
  Delay248/1 -> Mux141/2
  AddSub86/1 -> Mux85/3
  Delay555/1 -> Delay528/1, Relational124/1
  Delay535/1 -> Mux122/2
  Delay229/1 -> Mux105/1
  Delay468/1 -> Mux174/1
